simulink model "TransmissionController"  (R2026a)
settings: Solver=FixedStepAuto  StopTime=65  FixedStep=0.01
undefined symbols (not defined in the file): RangeSelected
libraries: simulink x26, sl_discontinuities x1
settings Model: DataDictionary=ETRS_data.sldd  Creator=macec  LastModifiedBy=Ved

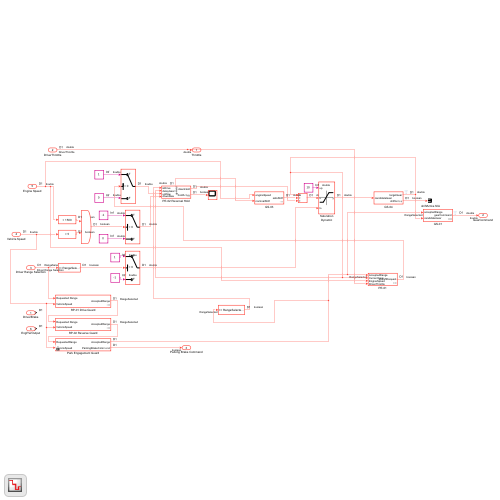
[thumbnail: Simulink's stored preview of the top-level diagram]
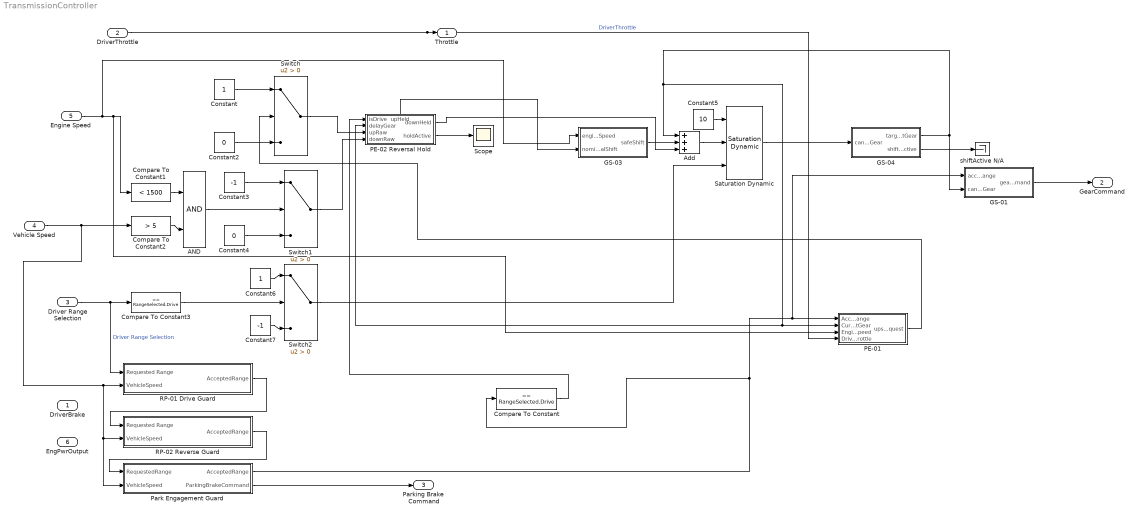
== system TransmissionController ==
  DriverBrake : Inport  OutDataTypeStr=double  PortDimensions=1
  DriverThrottle : Inport  Port=2  OutDataTypeStr=double  PortDimensions=1
  Driver Range Selection : Inport  Port=3  OutDataTypeStr=Enum: RangeSelected  PortDimensions=1
  Vehicle Speed : Inport  Port=4  OutDataTypeStr=double  PortDimensions=1
  Engine Speed : Inport  Port=5  OutDataTypeStr=double  PortDimensions=1
  EngPwrOutput : Inport  Port=6
  AND : Logic  IconShape=distinctive  AllPortsSameDT=off  OutDataTypeStr=boolean
  Add : Sum  Inputs=+++
  Compare To Constant : simulink/Logic and Bit Operations/Compare To Constant  relop===  const=RangeSelected.Drive  OutDataTypeStr=boolean
  Compare To Constant1 : simulink/Logic and Bit Operations/Compare To Constant  relop=<  const=1500  OutDataTypeStr=boolean
  Compare To Constant2 : simulink/Logic and Bit Operations/Compare To Constant  relop=>  const=5  OutDataTypeStr=boolean
  Compare To Constant3 : simulink/Logic and Bit Operations/Compare To Constant  relop===  const=RangeSelected.Drive  OutDataTypeStr=boolean
  Constant : Constant
  Constant2 : Constant  Value=0
  Constant3 : Constant  Value=-1
  Constant4 : Constant  Value=0
  Constant5 : Constant  Value=10
  Constant6 : Constant
  Constant7 : Constant  Value=-1
  GS-01 : Subsystem
  GS-03 : Subsystem
  GS-04 : Subsystem
  PE-01 : Subsystem
  PE-02 Reversal Hold : Subsystem
      settings: PortSchema="{\"entries\":[{\"content\":{\"sides\":[{\"content\":{\"connectorIds\":[\"In1\",\"In2\",\"In3\",\"In4\"]},\"type\":\"ConnectorPlacement.EquallySpacedRectSide\",\"uuid\":\"6e65c92f-9b0e-4c65-bd7f-8047c48f1be2\"},{\"content\":{\"connectorIds\":[\"Out1\",\"Out2\"],\"side\":\"RIGHT\"},\"type\":\"ConnectorPlacement.EquallySpacedRectSide\",\"uuid\":\"4f385b0c-417c-41ff-a848-cdf3ab5e0e25\"},{\"content\":{\"connectorIds\":[\"Out3\"],\"side\":\"TOP\"},\"type\":\"ConnectorPlacement.EquallySpacedRectSide\",\"uuid\":\"33776d86-75c0-4f20-bde1-77218aa26563\"}]},\"type\":\"ConnectorPlacement.EquallySpacedConnector\",\"uuid\":\"3a128240-7598-48df-bbc5-1501aee302e7\"}],\"packageUris\":[\"http://schema.mathworks.com/mf0/Connector/R2020b\"],\"version\":\"1.0\"}"
  Park Engagement Guard : Subsystem
  RP-01 Drive Guard : Subsystem
  RP-02 Reverse Guard : Subsystem
  Saturation Dynamic : sl_discontinuities/Saturation Dynamic  OutMin=[]  OutMax=[]  OutDataTypeStr=Inherit: Same as second input  OutDataType=fixdt(1, 16)  OutScaling=2^-10  DoSatur=off
      settings: LibrarySourceBlock=|
      | simulink/Discontinuities/Saturation
      | Dynamic
  Scope : Scope
  Switch : Switch  Criteria=u2 > Threshold  SaturateOnIntegerOverflow=off  InputSameDT=off
  Switch1 : Switch  Criteria=u2 > Threshold  SaturateOnIntegerOverflow=off  InputSameDT=off
  Switch2 : Switch  Criteria=u2 > Threshold  SaturateOnIntegerOverflow=off  InputSameDT=off
  shiftActive N/A : Terminator
  Throttle : Outport  OutDataTypeStr=double  PortDimensions=1
  GearCommand : Outport  Port=2  OutDataTypeStr=double  PortDimensions=1
  Parking Brake Command : Outport  Port=3  OutDataTypeStr=boolean  PortDimensions=1
  wires:
  Driver Range Selection/1 -> Compare To Constant3/1, RP-01 Drive Guard/1(Requested Range)  "Driver Range Selection"
  Engine Speed/1 -> Compare To Constant1/1, PE-01/3(EngineSpeed), GS-03/1(engineSpeed)
  PE-01/1(upshiftRequest) -> Switch/2
  Constant/1 -> Switch/1
  Constant2/1 -> Switch/3
  Constant3/1 -> Switch1/1
  Constant4/1 -> Switch1/3
  Compare To Constant2/1 -> AND/2
  AND/1 -> Switch1/2
  Compare To Constant1/1 -> AND/1
  Switch1/1 -> PE-02 Reversal Hold/4(downRaw)
  Switch/1 -> PE-02 Reversal Hold/3(upRaw)
  GS-04/1(targetGear) -> GS-01/2(candidateGear), Add/1, PE-02 Reversal Hold/2(delayGear), PE-01/2(CurrentGear)
  Constant5/1 -> Saturation Dynamic/1
  Add/1 -> Saturation Dynamic/2
  Constant6/1 -> Switch2/1
  Constant7/1 -> Switch2/3
  Switch2/1 -> Saturation Dynamic/3
  DriverThrottle/1 -> PE-01/4(DriverThrottle), Throttle/1  "DriverThrottle"
  Compare To Constant3/1 -> Switch2/2
  Vehicle Speed/1 -> Compare To Constant2/1, RP-01 Drive Guard/2(VehicleSpeed), RP-02 Reverse Guard/2(VehicleSpeed), Park Engagement Guard/2(VehicleSpeed)
  GS-01/1(gearCommand) -> GearCommand/1
  GS-03/1(safeShift) -> Add/2
  RP-01 Drive Guard/1(AcceptedRange) -> RP-02 Reverse Guard/1(Requested Range)
  RP-02 Reverse Guard/1(AcceptedRange) -> Park Engagement Guard/1(RequestedRange)
  Park Engagement Guard/1(AcceptedRange) -> PE-01/1(AcceptedRange), GS-01/1(acceptedRange), Compare To Constant/1
  Park Engagement Guard/2(ParkingBrakeCommand) -> Parking Brake Command/1
  Compare To Constant/1 -> PE-02 Reversal Hold/1(isDrive)
  PE-02 Reversal Hold/3(upHeld) -> GS-03/2(nominalShift)
  PE-02 Reversal Hold/1(downHeld) -> Add/3
  PE-02 Reversal Hold/2(holdActive) -> Scope/1
  Saturation Dynamic/1 -> GS-04/1(candidateGear)
  GS-04/2(shiftActive) -> shiftActive N/A/1

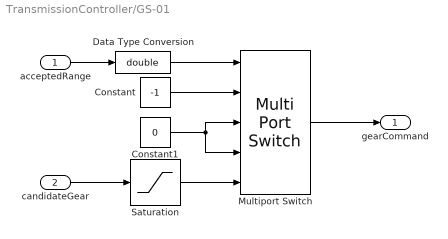
== system TransmissionController/GS-01 ==
  acceptedRange : Inport
  candidateGear : Inport  Port=2
  Constant : Constant  Value=-1
  Constant1 : Constant  Value=0
  Data Type Conversion : DataTypeConversion  OutDataTypeStr=double  SaturateOnIntegerOverflow=off  RndMeth=Floor
  Multiport Switch : MultiPortSwitch  DataPortOrder=Specify indices  Inputs=4  DataPortIndices={0,1,2,3}  SaturateOnIntegerOverflow=off  InputSameDT=off
  Saturation : Saturate  UpperLimit=10  LowerLimit=1
  gearCommand : Outport
  wires:
  candidateGear/1 -> Saturation/1
  Constant1/1 -> Multiport Switch/4, Multiport Switch/3
  Constant/1 -> Multiport Switch/2
  Saturation/1 -> Multiport Switch/5
  Multiport Switch/1 -> gearCommand/1
  acceptedRange/1 -> Data Type Conversion/1
  Data Type Conversion/1 -> Multiport Switch/1

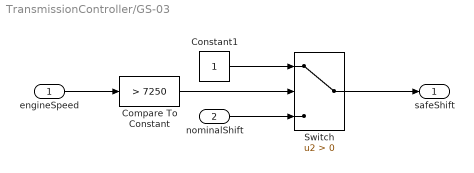
== system TransmissionController/GS-03 ==
  engineSpeed : Inport
  nominalShift : Inport  Port=2
  Compare To Constant : simulink/Logic and Bit Operations/Compare To Constant  relop=>  const=7250  OutDataTypeStr=boolean
  Constant1 : Constant
  Switch : Switch  Criteria=u2 > Threshold  SaturateOnIntegerOverflow=off  InputSameDT=off
  safeShift : Outport
  wires:
  engineSpeed/1 -> Compare To Constant/1
  Constant1/1 -> Switch/1
  nominalShift/1 -> Switch/3
  Switch/1 -> safeShift/1
  Compare To Constant/1 -> Switch/2

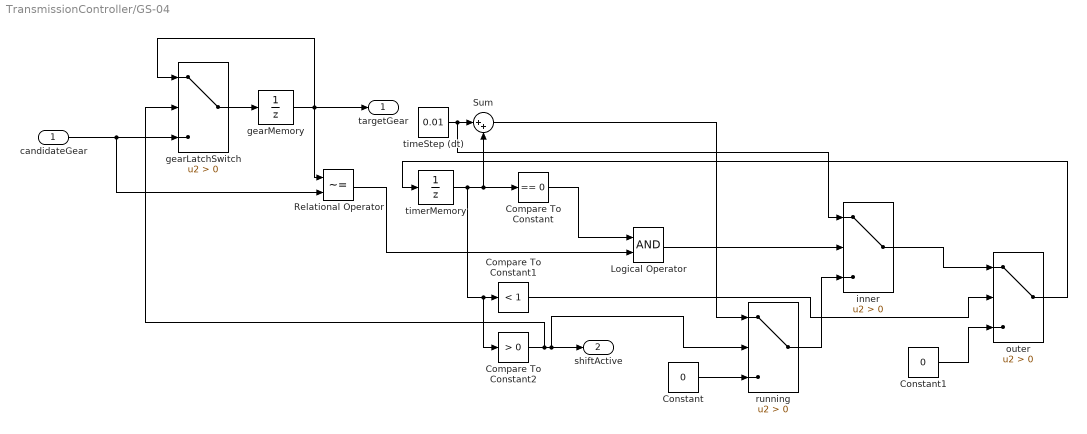
== system TransmissionController/GS-04 ==
  candidateGear : Inport
  Compare To Constant : simulink/Logic and Bit Operations/Compare To Constant  relop===  const=0  OutDataTypeStr=boolean
  Compare To Constant1 : simulink/Logic and Bit Operations/Compare To Constant  relop=<  const=1  OutDataTypeStr=boolean
  Compare To Constant2 : simulink/Logic and Bit Operations/Compare To Constant  relop=>  const=0  OutDataTypeStr=boolean
  Constant : Constant  Value=0
  Constant1 : Constant  Value=0
  Logical Operator : Logic  AllPortsSameDT=off  OutDataTypeStr=boolean
  Relational Operator : RelationalOperator  Operator=~=  OutDataTypeStr=boolean  RndMeth=Simplest  InputSameDT=off
  Sum : Sum  Inputs=|++
  gearLatchSwitch : Switch  Criteria=u2 > Threshold  SaturateOnIntegerOverflow=off  InputSameDT=off
  gearMemory : UnitDelay  InitialCondition=1  SampleTime=-1
  inner : Switch  Criteria=u2 > Threshold  SaturateOnIntegerOverflow=off  InputSameDT=off
  outer : Switch  Criteria=u2 > Threshold  SaturateOnIntegerOverflow=off  InputSameDT=off
  running : Switch  Criteria=u2 > Threshold  SaturateOnIntegerOverflow=off  InputSameDT=off
  timeStep (dt) : Constant  Value=0.01
  timerMemory : UnitDelay  SampleTime=-1
  targetGear : Outport
  shiftActive : Outport  Port=2
  wires:
  gearMemory/1 -> gearLatchSwitch/1, Relational Operator/1, targetGear/1
  candidateGear/1 -> Relational Operator/2, gearLatchSwitch/3
  timerMemory/1 -> Compare To Constant2/1, Compare To Constant1/1, Sum/2, Compare To Constant/1
  Compare To Constant/1 -> Logical Operator/1
  timeStep (dt)/1 -> inner/1, Sum/1
  Compare To Constant2/1 -> gearLatchSwitch/2, running/2, shiftActive/1
  Relational Operator/1 -> Logical Operator/2
  Logical Operator/1 -> inner/2
  running/1 -> inner/3
  Sum/1 -> running/1
  Constant/1 -> running/3
  Compare To Constant1/1 -> outer/2
  inner/1 -> outer/1
  Constant1/1 -> outer/3
  outer/1 -> timerMemory/1
  gearLatchSwitch/1 -> gearMemory/1

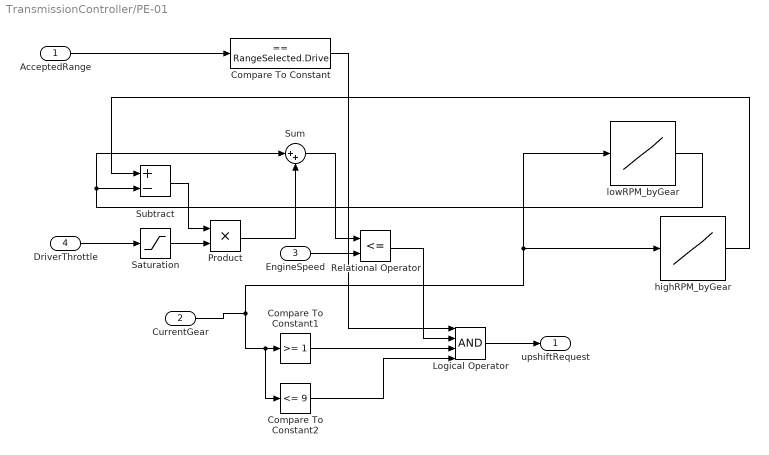
== system TransmissionController/PE-01 ==
  AcceptedRange : Inport
  CurrentGear : Inport  Port=2
  EngineSpeed : Inport  Port=3
  DriverThrottle : Inport  Port=4
  Compare To Constant : simulink/Logic and Bit Operations/Compare To Constant  relop===  const=RangeSelected.Drive  OutDataTypeStr=boolean
  Compare To Constant1 : simulink/Logic and Bit Operations/Compare To Constant  relop=>=  const=1  OutDataTypeStr=uint8
  Compare To Constant2 : simulink/Logic and Bit Operations/Compare To Constant  relop=<=  const=9  OutDataTypeStr=uint8
  Logical Operator : Logic  Inputs=4  AllPortsSameDT=off  OutDataTypeStr=boolean
  Product : Product
  Relational Operator : RelationalOperator  Operator=<=  OutDataTypeStr=boolean  RndMeth=Simplest  InputSameDT=off
  Saturation : Saturate  UpperLimit=1.0  LowerLimit=0.0
  Subtract : Sum  Inputs=+-
  Sum : Sum  Inputs=|++
  highRPM_byGear : Lookup_n-D  NumberOfTableDimensions=1  BreakpointsForDimension1=[1 2 3 4 5 6 7 8 9]  Table=[6000 6000 6000 6000 6000 6000 6000 6000 6000]  InternalRulePriority=Speed  RndMeth=Simplest
  lowRPM_byGear : Lookup_n-D  NumberOfTableDimensions=1  BreakpointsForDimension1=[1 2 3 4 5 6 7 8 9]  Table=[4500 4500 4500 4500 4500 4500 4500 4500 4500]  InternalRulePriority=Speed  RndMeth=Simplest
  upshiftRequest : Outport
  wires:
  Saturation/1 -> Product/2
  Subtract/1 -> Product/1
  DriverThrottle/1 -> Saturation/1
  lowRPM_byGear/1 -> Sum/1, Subtract/2
  highRPM_byGear/1 -> Subtract/1
  Product/1 -> Sum/2
  Sum/1 -> Relational Operator/1
  EngineSpeed/1 -> Relational Operator/2
  AcceptedRange/1 -> Compare To Constant/1
  CurrentGear/1 -> highRPM_byGear/1, lowRPM_byGear/1, Compare To Constant2/1, Compare To Constant1/1
  Compare To Constant1/1 -> Logical Operator/3
  Relational Operator/1 -> Logical Operator/2
  Compare To Constant/1 -> Logical Operator/1
  Logical Operator/1 -> upshiftRequest/1
  Compare To Constant2/1 -> Logical Operator/4

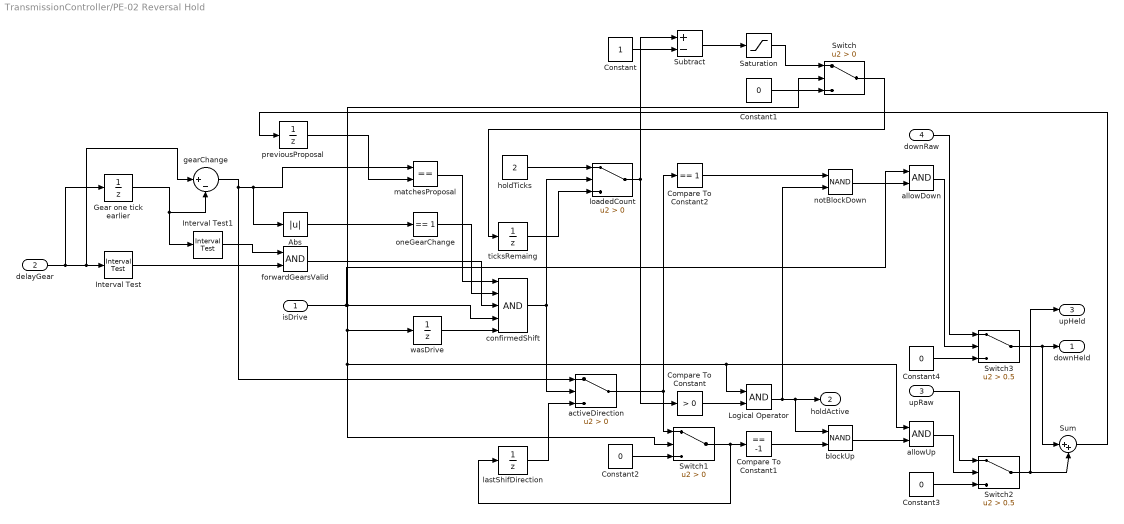
== system TransmissionController/PE-02 Reversal Hold ==
  isDrive : Inport
  delayGear : Inport  Port=2
  upRaw : Inport  Port=3
  downRaw : Inport  Port=4
  Abs : Abs  SaturateOnIntegerOverflow=off
  Compare To Constant : simulink/Logic and Bit Operations/Compare To Constant  relop=>  const=0  OutDataTypeStr=boolean
  Compare To Constant1 : simulink/Logic and Bit Operations/Compare To Constant  relop===  const=-1  OutDataTypeStr=boolean
  Compare To Constant2 : simulink/Logic and Bit Operations/Compare To Constant  relop===  const=1  OutDataTypeStr=boolean
  Constant : Constant
  Constant{1..4} (4 alike) : Constant  Value=0
  Gear one tick earlier : UnitDelay  SampleTime=-1
  Interval Test : simulink/Logic and Bit Operations/Interval Test  IntervalClosedRight=on  uplimit=10  IntervalClosedLeft=on  lowlimit=1  OutDataTypeStr=boolean
  Interval Test1 : simulink/Logic and Bit Operations/Interval Test  IntervalClosedRight=on  uplimit=10  IntervalClosedLeft=on  lowlimit=1  OutDataTypeStr=boolean
  Logical Operator : Logic  AllPortsSameDT=off  OutDataTypeStr=boolean
  Saturation : Saturate  UpperLimit=2  LowerLimit=0  OutDataTypeStr=uint8
  Subtract : Sum  Inputs=+-
  Sum : Sum  Inputs=|++
  Switch : Switch  Criteria=u2 > Threshold  SaturateOnIntegerOverflow=off  InputSameDT=off
  Switch1 : Switch  Criteria=u2 > Threshold  SaturateOnIntegerOverflow=off  InputSameDT=off
  Switch2 : Switch  Criteria=u2 > Threshold  Threshold=0.5  SaturateOnIntegerOverflow=off  InputSameDT=off
  Switch3 : Switch  Criteria=u2 > Threshold  Threshold=0.5  SaturateOnIntegerOverflow=off  InputSameDT=off
  activeDirection : Switch  Criteria=u2 > Threshold  SaturateOnIntegerOverflow=off  InputSameDT=off
  allowDown : Logic  AllPortsSameDT=off  OutDataTypeStr=boolean
  allowUp : Logic  AllPortsSameDT=off  OutDataTypeStr=boolean
  blockUp : Logic  Operator=NAND  AllPortsSameDT=off  OutDataTypeStr=boolean
  confirmedShift : Logic  Inputs=5  AllPortsSameDT=off  OutDataTypeStr=boolean
  forwardGearsValid : Logic  AllPortsSameDT=off  OutDataTypeStr=boolean
  gearChange : Sum  Inputs=|+-
  holdTicks : Constant  Value=2
  lastShifDirection : UnitDelay  SampleTime=-1
  loadedCount : Switch  Criteria=u2 > Threshold  SaturateOnIntegerOverflow=off  InputSameDT=off
  matchesProposal : RelationalOperator  Operator===  OutDataTypeStr=boolean  RndMeth=Simplest  InputSameDT=off
  notBlockDown : Logic  Operator=NAND  AllPortsSameDT=off  OutDataTypeStr=boolean
  oneGearChange : simulink/Logic and Bit Operations/Compare To Constant  relop===  const=1  OutDataTypeStr=boolean
  previousProposal : UnitDelay  SampleTime=-1
  ticksRemaing : UnitDelay  SampleTime=-1
  wasDrive : UnitDelay  SampleTime=-1
  downHeld : Outport
  holdActive : Outport  Port=2
  upHeld : Outport  Port=3
  wires:
  Constant/1 -> Subtract/2
  Abs/1 -> oneGearChange/1
  downRaw/1 -> Switch3/1
  Interval Test1/1 -> forwardGearsValid/1
  Compare To Constant2/1 -> notBlockDown/1
  delayGear/1 -> Interval Test/1, gearChange/1, Gear one tick earlier/1
  forwardGearsValid/1 -> confirmedShift/3
  previousProposal/1 -> matchesProposal/2
  Sum/1 -> previousProposal/1
  notBlockDown/1 -> allowDown/2
  Gear one tick earlier/1 -> gearChange/2, Interval Test1/1
  Interval Test/1 -> forwardGearsValid/2
  gearChange/1 -> matchesProposal/1, Abs/1, activeDirection/1
  Switch2/1 -> Sum/2, upHeld/1
  isDrive/1 -> confirmedShift/4, wasDrive/1, allowUp/1, Logical Operator/1, Switch1/2, Switch/2, allowDown/1
  matchesProposal/1 -> confirmedShift/1
  oneGearChange/1 -> confirmedShift/2
  wasDrive/1 -> confirmedShift/5
  holdTicks/1 -> loadedCount/1
  Constant2/1 -> Switch1/3
  ticksRemaing/1 -> loadedCount/3
  confirmedShift/1 -> loadedCount/2, activeDirection/2
  lastShifDirection/1 -> activeDirection/3
  loadedCount/1 -> Subtract/1, Compare To Constant/1
  activeDirection/1 -> Switch1/1, Compare To Constant2/1
  Subtract/1 -> Saturation/1
  Compare To Constant/1 -> Logical Operator/2
  Switch1/1 -> lastShifDirection/1, Compare To Constant1/1
  upRaw/1 -> Switch2/1
  Saturation/1 -> Switch/1
  Constant1/1 -> Switch/3
  Logical Operator/1 -> blockUp/1, holdActive/1, notBlockDown/2
  Compare To Constant1/1 -> blockUp/2
  Switch/1 -> ticksRemaing/1
  blockUp/1 -> allowUp/2
  allowDown/1 -> Switch3/2
  Switch3/1 -> downHeld/1, Sum/1
  Constant4/1 -> Switch3/3
  allowUp/1 -> Switch2/2
  Constant3/1 -> Switch2/3

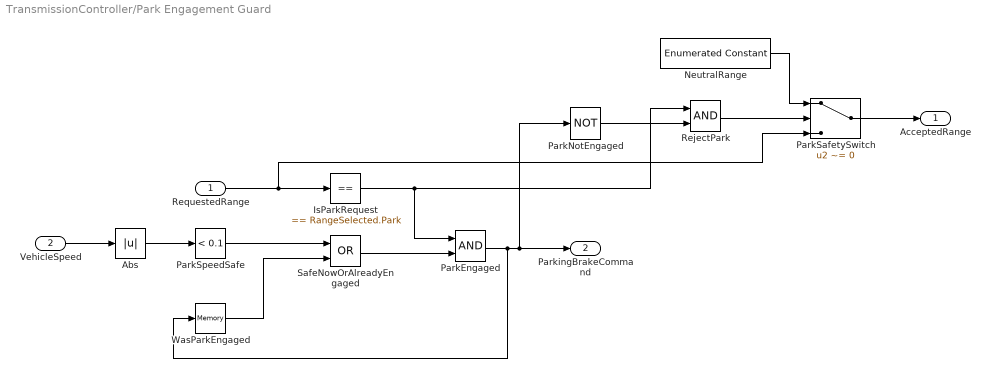
== system TransmissionController/Park Engagement Guard ==
  RequestedRange : Inport
  VehicleSpeed : Inport  Port=2
  Abs : Abs  SaturateOnIntegerOverflow=off
  IsParkRequest : simulink/Logic and Bit Operations/Compare To Constant  relop===  const=RangeSelected.Park  OutDataTypeStr=boolean
  NeutralRange : simulink/Sources/Enumerated Constant  OutDataTypeStr=Enum: RangeSelected  Value=RangeSelected.Neutral  SampleTime=inf
  ParkEngaged : Logic  AllPortsSameDT=off  OutDataTypeStr=boolean
  ParkNotEngaged : Logic  Operator=NOT  AllPortsSameDT=off  OutDataTypeStr=boolean
  ParkSafetySwitch : Switch  Criteria=u2 ~= 0  SaturateOnIntegerOverflow=off  InputSameDT=off
  ParkSpeedSafe : simulink/Logic and Bit Operations/Compare To Constant  relop=<  const=0.1  OutDataTypeStr=boolean
  RejectPark : Logic  AllPortsSameDT=off  OutDataTypeStr=boolean
  SafeNowOrAlreadyEngaged : Logic  Operator=OR  AllPortsSameDT=off  OutDataTypeStr=boolean
  WasParkEngaged : Memory
  AcceptedRange : Outport
  ParkingBrakeCommand : Outport  Port=2
  wires:
  ParkEngaged/1 -> ParkNotEngaged/1, ParkingBrakeCommand/1, WasParkEngaged/1
  SafeNowOrAlreadyEngaged/1 -> ParkEngaged/2
  RequestedRange/1 -> ParkSafetySwitch/3, IsParkRequest/1
  VehicleSpeed/1 -> Abs/1
  Abs/1 -> ParkSpeedSafe/1
  WasParkEngaged/1 -> SafeNowOrAlreadyEngaged/2
  IsParkRequest/1 -> RejectPark/1, ParkEngaged/1
  ParkSpeedSafe/1 -> SafeNowOrAlreadyEngaged/1
  ParkNotEngaged/1 -> RejectPark/2
  NeutralRange/1 -> ParkSafetySwitch/1
  RejectPark/1 -> ParkSafetySwitch/2
  ParkSafetySwitch/1 -> AcceptedRange/1

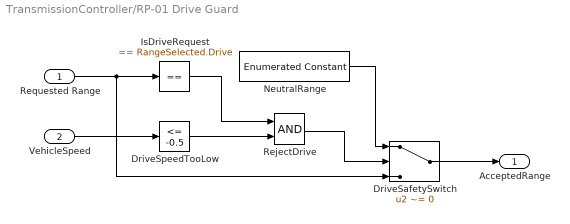
== system TransmissionController/RP-01 Drive Guard ==
  Requested Range : Inport
  VehicleSpeed : Inport  Port=2
  DriveSafetySwitch : Switch  Criteria=u2 ~= 0  SaturateOnIntegerOverflow=off  InputSameDT=off
  DriveSpeedTooLow : simulink/Logic and Bit Operations/Compare To Constant  relop=<=  const=-0.5  OutDataTypeStr=boolean
  IsDriveRequest : simulink/Logic and Bit Operations/Compare To Constant  relop===  const=RangeSelected.Drive  OutDataTypeStr=boolean
  NeutralRange : simulink/Sources/Enumerated Constant  OutDataTypeStr=Enum: RangeSelected  Value=RangeSelected.Neutral  SampleTime=inf
  RejectDrive : Logic  AllPortsSameDT=off  OutDataTypeStr=boolean
  AcceptedRange : Outport  OutDataTypeStr=Enum: RangeSelected
  wires:
  NeutralRange/1 -> DriveSafetySwitch/1
  VehicleSpeed/1 -> DriveSpeedTooLow/1
  Requested Range/1 -> DriveSafetySwitch/3, IsDriveRequest/1
  IsDriveRequest/1 -> RejectDrive/1
  RejectDrive/1 -> DriveSafetySwitch/2
  DriveSpeedTooLow/1 -> RejectDrive/2
  DriveSafetySwitch/1 -> AcceptedRange/1

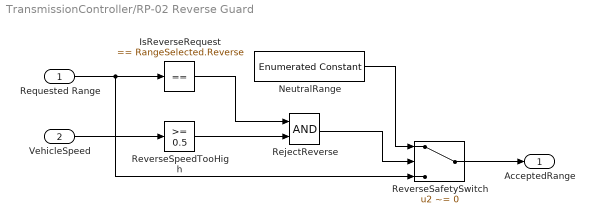
== system TransmissionController/RP-02 Reverse Guard ==
  Requested Range : Inport
  VehicleSpeed : Inport  Port=2
  IsReverseRequest : simulink/Logic and Bit Operations/Compare To Constant  relop===  const=RangeSelected.Reverse  OutDataTypeStr=boolean
  NeutralRange : simulink/Sources/Enumerated Constant  OutDataTypeStr=Enum: RangeSelected  Value=RangeSelected.Neutral  SampleTime=inf
  RejectReverse : Logic  AllPortsSameDT=off  OutDataTypeStr=boolean
  ReverseSafetySwitch : Switch  Criteria=u2 ~= 0  SaturateOnIntegerOverflow=off  InputSameDT=off
  ReverseSpeedTooHigh : simulink/Logic and Bit Operations/Compare To Constant  relop=>=  const=0.5  OutDataTypeStr=boolean
  AcceptedRange : Outport
  wires:
  Requested Range/1 -> ReverseSafetySwitch/3, IsReverseRequest/1
  IsReverseRequest/1 -> RejectReverse/1
  VehicleSpeed/1 -> ReverseSpeedTooHigh/1
  RejectReverse/1 -> ReverseSafetySwitch/2
  ReverseSpeedTooHigh/1 -> RejectReverse/2
  NeutralRange/1 -> ReverseSafetySwitch/1
  ReverseSafetySwitch/1 -> AcceptedRange/1
